simulink model "Step"  (R2018b)
settings: Solver=FixedStepDiscrete  StartTime=0.0  StopTime=10.0  RelTol=1e-3
libraries: simulink x5, vrlib x2
settings Model: Creator=taste  LastModifiedBy=taste
settings DataIOCC: SaveOutput=off  SignalLogging=off  SaveTime=off  ReturnWorkspaceOutputs=on
settings OptimizationCC: DefaultParameterBehavior=Inlined  EnhancedBackFolding=on  PassReuseOutputArgsAs=Individual arguments  ZeroExternalMemoryAtStartup=off  ZeroInternalMemoryAtStartup=off  OptimizeBlockOrder=speed  DifferentSizesBufferReuse=on  OptimizationCustomize=off
settings DebuggingCC: ParameterTunabilityLossMsg=error
settings SFSimCC: MATLABDynamicMemAlloc=off
settings RTWCC: SystemTargetFile=ert.tlc  TemplateMakefile=ert_default_tmf  PostCodeGenCommand=packNGo(buildInfo);
settings CodeAppCC: ForceParamTrailComments=on  IgnoreCustomStorageClasses=off  OperatorAnnotations=on  SimulinkDataObjDesc=on  SFDataObjDesc=on  InsertBlockDesc=on
settings ERTTargetCC: TargetLangStandard=C99 (ISO)  GenerateSampleERTMain=on  InlinedParameterPlacement=NonHierarchical  ERTCustomFileTemplate=example_file_process.tlc

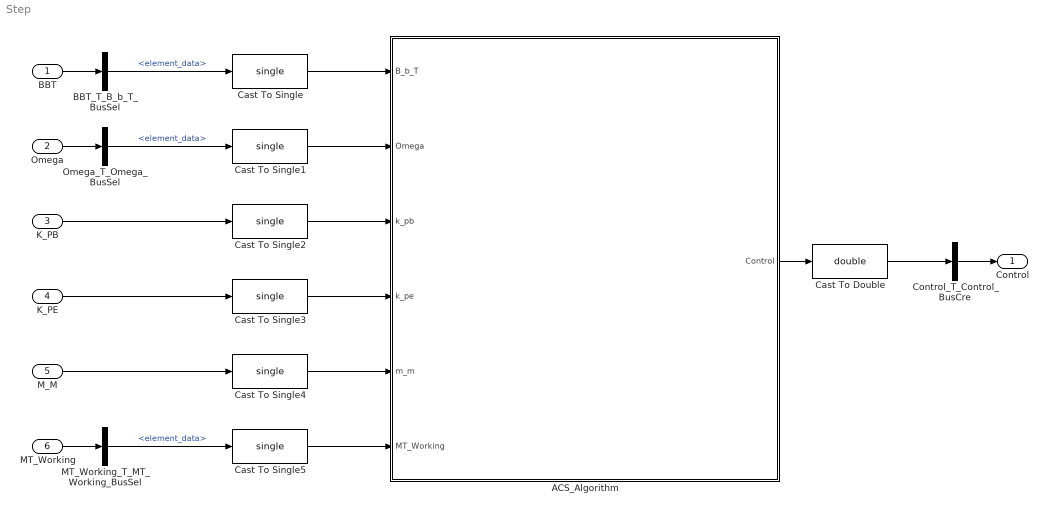
== system Step ==
  BBT : Inport  OutDataTypeStr=Bus: T_B_b_T  BusOutputAsStruct=on
  Omega : Inport  Port=2  OutDataTypeStr=Bus: T_Omega  BusOutputAsStruct=on
  K_PB : Inport  Port=3  OutDataTypeStr=T_Float  BusOutputAsStruct=on
  K_PE : Inport  Port=4  OutDataTypeStr=T_Float  BusOutputAsStruct=on
  M_M : Inport  Port=5  OutDataTypeStr=T_Float  BusOutputAsStruct=on
  MT_Working : Inport  Port=6  OutDataTypeStr=Bus: T_MT_Working  BusOutputAsStruct=on
  ACS_Algorithm : Subsystem
  BBT_T_B_b_T_BusSel : BusSelector  OutputSignals=element_data
  Cast To Double : DataTypeConversion  OutDataTypeStr=double
  Cast To Single{,1..5} (6 alike) : DataTypeConversion  OutDataTypeStr=single
  Control_T_Control_BusCre : BusCreator  Inputs=1  OutDataTypeStr=Bus: T_Control  NonVirtualBus=on
  MT_Working_T_MT_Working_BusSel : BusSelector  OutputSignals=element_data
  Omega_T_Omega_BusSel : BusSelector  OutputSignals=element_data
  Control : Outport  OutDataTypeStr=Bus: T_Control  BusOutputAsStruct=on
  wires:
  ACS_Algorithm/1(Control) -> Cast To Double/1
  Cast To Single/1 -> ACS_Algorithm/1(B_b_T)
  Cast To Single1/1 -> ACS_Algorithm/2(Omega)
  Cast To Single2/1 -> ACS_Algorithm/3(k_pb)
  Cast To Single3/1 -> ACS_Algorithm/4(k_pe)
  Cast To Single4/1 -> ACS_Algorithm/5(m_m)
  Cast To Single5/1 -> ACS_Algorithm/6(MT_Working)
  BBT/1 -> BBT_T_B_b_T_BusSel/1
  Omega/1 -> Omega_T_Omega_BusSel/1
  MT_Working/1 -> MT_Working_T_MT_Working_BusSel/1
  Control_T_Control_BusCre/1 -> Control/1
  BBT_T_B_b_T_BusSel/1 -> Cast To Single/1  "<element_data>"
  Omega_T_Omega_BusSel/1 -> Cast To Single1/1  "<element_data>"
  K_PB/1 -> Cast To Single2/1
  K_PE/1 -> Cast To Single3/1
  M_M/1 -> Cast To Single4/1
  MT_Working_T_MT_Working_BusSel/1 -> Cast To Single5/1  "<element_data>"
  Cast To Double/1 -> Control_T_Control_BusCre/1

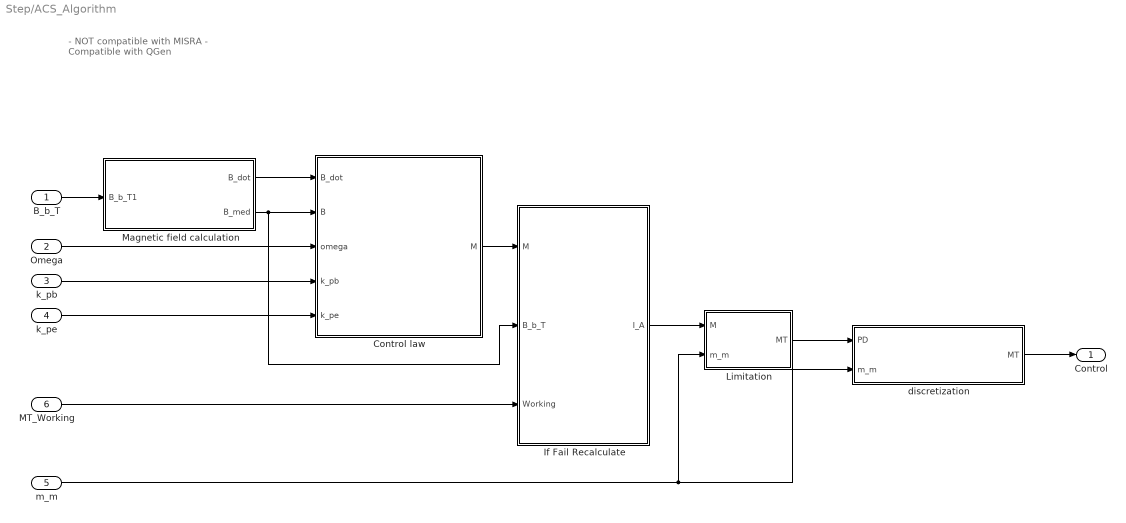
== system Step/ACS_Algorithm ==
  note: - NOT compatible with MISRA
      | - Compatible with QGen
  B_b_T : Inport  PortDimensions=15
  Omega : Inport  Port=2  PortDimensions=3
  k_pb : Inport  Port=3  PortDimensions=1
  k_pe : Inport  Port=4  PortDimensions=1
  m_m : Inport  Port=5  PortDimensions=1
  MT_Working : Inport  Port=6  PortDimensions=3
  Control law : Subsystem
  If Fail Recalculate : Subsystem
  Limitation : Subsystem
  Magnetic field calculation : Subsystem
  discretization : Subsystem
  Control : Outport  VectorParamsAs1DForOutWhenUnconnected=off
  wires:
  k_pb/1 -> Control law/4(k_pb)
  Magnetic field calculation/2(B_med) -> If Fail Recalculate/2(B_b_T), Control law/2(B)
  Omega/1 -> Control law/3(omega)
  Limitation/1(MT) -> discretization/1(PD)
  k_pe/1 -> Control law/5(k_pe)
  B_b_T/1 -> Magnetic field calculation/1(B_b_T1)
  If Fail Recalculate/1(I_A) -> Limitation/1(M)
  discretization/1(MT) -> Control/1
  Magnetic field calculation/1(B_dot) -> Control law/1(B_dot)
  m_m/1 -> Limitation/2(m_m), discretization/2(m_m)
  MT_Working/1 -> If Fail Recalculate/3(Working)
  Control law/1(M) -> If Fail Recalculate/1(M)

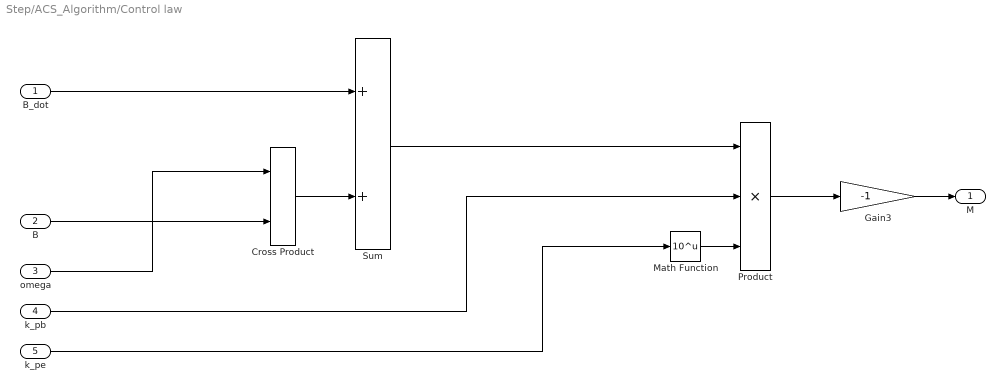
== system Step/ACS_Algorithm/Control law ==
  B_dot : Inport
  B : Inport  Port=2
  omega : Inport  Port=3
  k_pb : Inport  Port=4
  k_pe : Inport  Port=5
  Cross Product : vrlib/Utilities/Cross Product
  Gain3 : Gain  Gain=-1
  Math Function : Math  Operator=10^u  SaturateOnIntegerOverflow=on
  Product : Product  Inputs=3
  Sum : Sum  Inputs=2
  M : Outport  VectorParamsAs1DForOutWhenUnconnected=off
  wires:
  B/1 -> Cross Product/2
  Gain3/1 -> M/1
  Sum/1 -> Product/1
  B_dot/1 -> Sum/1
  Cross Product/1 -> Sum/2
  Product/1 -> Gain3/1
  Math Function/1 -> Product/3
  k_pb/1 -> Product/2
  k_pe/1 -> Math Function/1
  omega/1 -> Cross Product/1

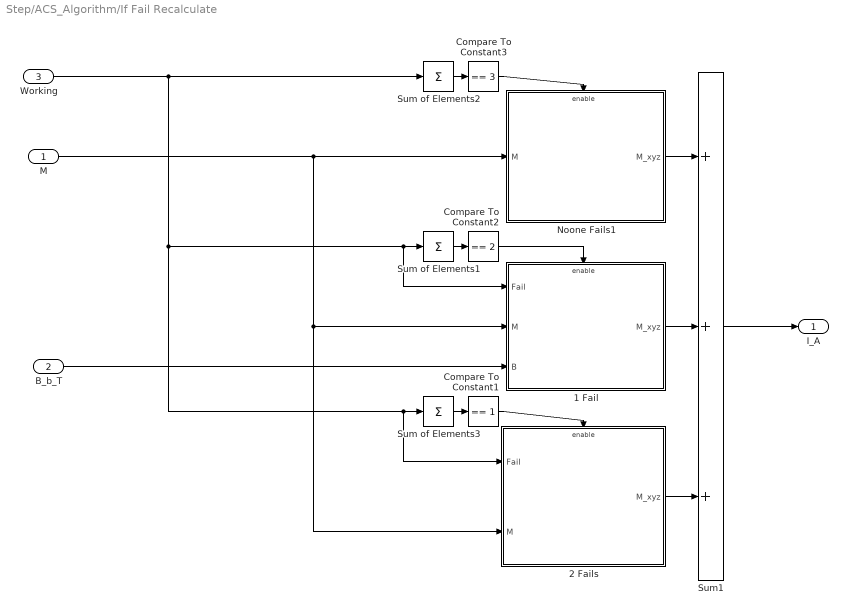
== system Step/ACS_Algorithm/If Fail Recalculate ==
  M : Inport
  B_b_T : Inport  Port=2
  Working : Inport  Port=3
  1 Fail : Subsystem
  2 Fails : Subsystem
  Compare To Constant1 : simulink/Logic and Bit Operations/Compare To Constant  relop===  const=1  OutDataTypeStr=uint8  ZeroCross=off
  Compare To Constant2 : simulink/Logic and Bit Operations/Compare To Constant  relop===  const=2  OutDataTypeStr=uint8  ZeroCross=off
  Compare To Constant3 : simulink/Logic and Bit Operations/Compare To Constant  relop===  const=3  OutDataTypeStr=uint8  ZeroCross=off
  Noone Fails1 : Subsystem
  Sum of Elements1 : Sum  Inputs=+
  Sum of Elements2 : Sum  Inputs=+
  Sum of Elements3 : Sum  Inputs=+
  Sum1 : Sum  Inputs=3
  I_A : Outport  VectorParamsAs1DForOutWhenUnconnected=off
  wires:
  Compare To Constant1/1 -> 2 Fails/Enable
  2 Fails/1(M_xyz) -> Sum1/3
  Sum of Elements3/1 -> Compare To Constant1/1
  Sum of Elements2/1 -> Compare To Constant3/1
  Sum of Elements1/1 -> Compare To Constant2/1
  M/1 -> 2 Fails/2(M), 1 Fail/2(M), Noone Fails1/1(M)
  Compare To Constant2/1 -> 1 Fail/Enable
  Compare To Constant3/1 -> Noone Fails1/Enable
  1 Fail/1(M_xyz) -> Sum1/2
  Noone Fails1/1(M_xyz) -> Sum1/1
  B_b_T/1 -> 1 Fail/3(B)
  Working/1 -> Sum of Elements2/1, 2 Fails/1(Fail), Sum of Elements3/1, 1 Fail/1(Fail), Sum of Elements1/1
  Sum1/1 -> I_A/1

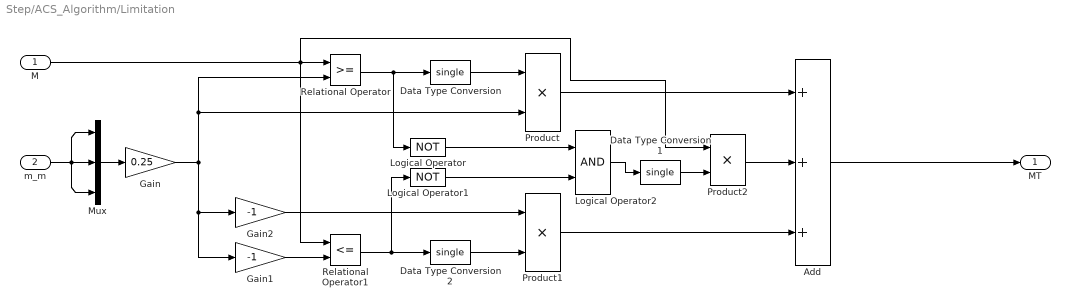
== system Step/ACS_Algorithm/Limitation ==
  M : Inport
  m_m : Inport  Port=2
  Add : Sum  Inputs=3
  Data Type Conversion : DataTypeConversion  OutDataTypeStr=single
  Data Type Conversion1 : DataTypeConversion  OutDataTypeStr=single
  Data Type Conversion2 : DataTypeConversion  OutDataTypeStr=single
  Gain : Gain  Gain=0.25
  Gain1 : Gain  Gain=-1
  Gain2 : Gain  Gain=-1
  Logical Operator : Logic  Operator=NOT  AllPortsSameDT=off  OutDataTypeStr=boolean
  Logical Operator1 : Logic  Operator=NOT  AllPortsSameDT=off  OutDataTypeStr=boolean
  Logical Operator2 : Logic  AllPortsSameDT=off  OutDataTypeStr=boolean
  Mux : Mux  Inputs=3
  Product : Product
  Product1 : Product
  Product2 : Product
  Relational Operator : RelationalOperator  OutDataTypeStr=boolean  RndMeth=Nearest
  Relational Operator1 : RelationalOperator  Operator=<=  OutDataTypeStr=boolean  RndMeth=Nearest
  MT : Outport  VectorParamsAs1DForOutWhenUnconnected=off
  wires:
  M/1 -> Product2/1, Relational Operator1/1, Relational Operator/1
  m_m/1 -> Mux/3, Mux/1, Mux/2
  Gain/1 -> Relational Operator/2, Product/2, Gain2/1, Gain1/1
  Gain1/1 -> Relational Operator1/2
  Relational Operator/1 -> Logical Operator/1, Data Type Conversion/1
  Relational Operator1/1 -> Logical Operator1/1, Data Type Conversion2/1
  Logical Operator/1 -> Logical Operator2/1
  Logical Operator1/1 -> Logical Operator2/2
  Logical Operator2/1 -> Data Type Conversion1/1
  Product/1 -> Add/1
  Product2/1 -> Add/2
  Product1/1 -> Add/3
  Gain2/1 -> Product1/1
  Mux/1 -> Gain/1
  Add/1 -> MT/1
  Data Type Conversion/1 -> Product/1
  Data Type Conversion1/1 -> Product2/2
  Data Type Conversion2/1 -> Product1/2

== system Step/ACS_Algorithm/Magnetic field calculation ==
  B_b_T1 : Inport
  Derivative : Subsystem
  Media : Subsystem
  B_dot : Outport  VectorParamsAs1DForOutWhenUnconnected=off
  B_med : Outport  Port=2  VectorParamsAs1DForOutWhenUnconnected=off
  wires:
  B_b_T1/1 -> Derivative/1(In1), Media/1(B_b_T_1s)
  Media/1(B_b_T_1s_m) -> B_med/1
  Derivative/1(B_dot) -> B_dot/1

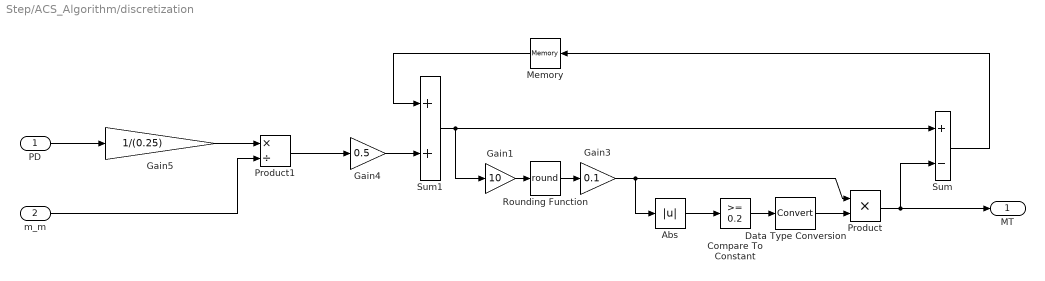
== system Step/ACS_Algorithm/discretization ==
  PD : Inport
  m_m : Inport  Port=2
  Abs : Abs
  Compare To Constant : simulink/Logic and Bit Operations/Compare To Constant  relop=>=  const=0.2  OutDataTypeStr=uint8  ZeroCross=off
  Data Type Conversion : DataTypeConversion
  Gain1 : Gain  Gain=10
  Gain3 : Gain  Gain=0.1
  Gain4 : Gain  Gain=0.5
  Gain5 : Gain  Gain=1/(0.25)
  Memory : Memory  InheritSampleTime=on
  Product : Product  RndMeth=Zero
  Product1 : Product  Inputs=*/  RndMeth=Zero
  Rounding Function : Rounding  Operator=round
  Sum : Sum  Inputs=+-
  Sum1 : Sum  Inputs=2
  MT : Outport  VectorParamsAs1DForOutWhenUnconnected=off
  wires:
  Rounding Function/1 -> Gain3/1
  Gain1/1 -> Rounding Function/1
  Sum/1 -> Memory/1
  Sum1/1 -> Gain1/1, Sum/1
  Gain3/1 -> Abs/1, Product/1
  Compare To Constant/1 -> Data Type Conversion/1
  Data Type Conversion/1 -> Product/2
  Abs/1 -> Compare To Constant/1
  PD/1 -> Gain5/1
  Product/1 -> MT/1, Sum/2
  Memory/1 -> Sum1/1
  Gain4/1 -> Sum1/2
  Gain5/1 -> Product1/1
  Product1/1 -> Gain4/1
  m_m/1 -> Product1/2

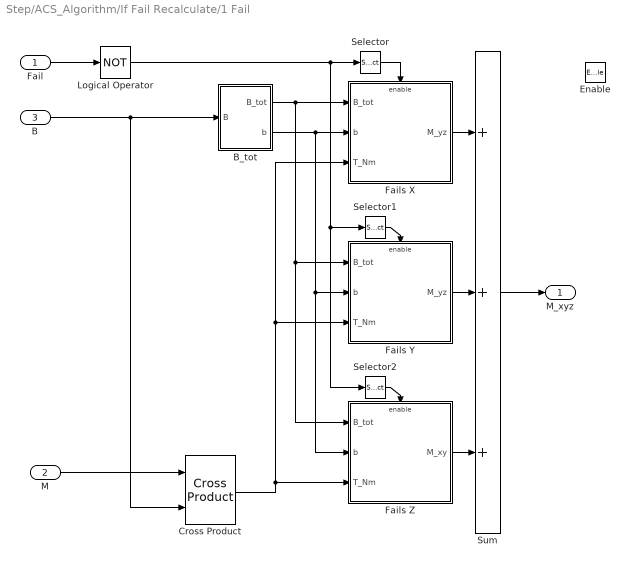
== system Step/ACS_Algorithm/If Fail Recalculate/1 Fail ==
  Fail : Inport
  M : Inport  Port=2
  B : Inport  Port=3
  Enable : EnablePort
  B_tot : Subsystem
  Cross Product : vrlib/Utilities/Cross Product
  Fails X : Subsystem
  Fails Y : Subsystem
  Fails Z : Subsystem
  Logical Operator : Logic  Operator=NOT  AllPortsSameDT=off  OutDataTypeStr=boolean
  Selector : Selector  InputPortWidth=3  IndexOptions=Index vector (dialog)  Indices=[1]  OutputSizes=1
  Selector1 : Selector  InputPortWidth=3  IndexOptions=Index vector (dialog)  Indices=[2]  OutputSizes=1
  Selector2 : Selector  InputPortWidth=3  IndexOptions=Index vector (dialog)  Indices=[3]  OutputSizes=1
  Sum : Sum  Inputs=3
  M_xyz : Outport  VectorParamsAs1DForOutWhenUnconnected=off
  wires:
  Sum/1 -> M_xyz/1
  M/1 -> Cross Product/1
  B/1 -> Cross Product/2, B_tot/1(B)
  B_tot/1(B_tot) -> Fails X/1(B_tot), Fails Y/1(B_tot), Fails Z/1(B_tot)
  B_tot/2(b) -> Fails Y/2(b), Fails Z/2(b), Fails X/2(b)
  Cross Product/1 -> Fails X/3(T_Nm), Fails Y/3(T_Nm), Fails Z/3(T_Nm)
  Fails X/1(M_yz) -> Sum/1
  Fails Y/1(M_yz) -> Sum/2
  Fails Z/1(M_xy) -> Sum/3
  Selector/1 -> Fails X/Enable
  Selector1/1 -> Fails Y/Enable
  Selector2/1 -> Fails Z/Enable
  Fail/1 -> Logical Operator/1
  Logical Operator/1 -> Selector/1, Selector1/1, Selector2/1

== system Step/ACS_Algorithm/If Fail Recalculate/2 Fails ==
  Fail : Inport
  M : Inport  Port=2
  Enable : EnablePort
  Demux1 : Demux  Outputs=3
  Demux3 : Demux  Outputs=3
  Mux : Mux  Inputs=3
  Product : Product  RndMeth=Zero
  Product1 : Product  RndMeth=Zero
  Product2 : Product  RndMeth=Zero
  M_xyz : Outport  VectorParamsAs1DForOutWhenUnconnected=off
  wires:
  Mux/1 -> M_xyz/1
  M/1 -> Demux3/1
  Product2/1 -> Mux/3
  Product1/1 -> Mux/2
  Product/1 -> Mux/1
  Demux3/1 -> Product/1
  Demux3/2 -> Product1/1
  Demux3/3 -> Product2/1
  Demux1/3 -> Product2/2
  Demux1/2 -> Product1/2
  Fail/1 -> Demux1/1
  Demux1/1 -> Product/2

== system Step/ACS_Algorithm/If Fail Recalculate/Noone Fails1 ==
  M : Inport
  Enable : EnablePort
  M_xyz : Outport  VectorParamsAs1DForOutWhenUnconnected=off
  wires:
  M/1 -> M_xyz/1

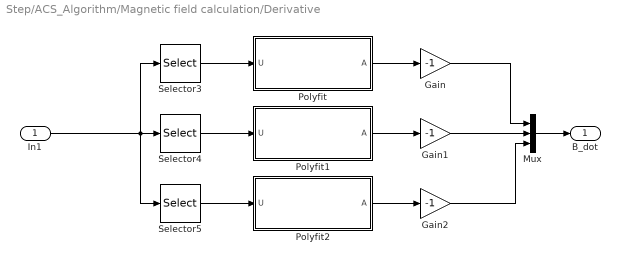
== system Step/ACS_Algorithm/Magnetic field calculation/Derivative ==
  In1 : Inport
  Gain : Gain  Gain=-1
  Gain1 : Gain  Gain=-1
  Gain2 : Gain  Gain=-1
  Mux : Mux  Inputs=3
  Polyfit : Subsystem
  Polyfit1 : Subsystem
  Polyfit2 : Subsystem
  Selector3 : Selector  InputPortWidth=15  IndexOptions=Index vector (dialog)  Indices=[1 4 7 10 13]  OutputSizes=1
  Selector4 : Selector  InputPortWidth=15  IndexOptions=Index vector (dialog)  Indices=[2 5 8 11 14]  OutputSizes=1
  Selector5 : Selector  InputPortWidth=15  IndexOptions=Index vector (dialog)  Indices=[3 6 9 12 15]  OutputSizes=1
  B_dot : Outport  VectorParamsAs1DForOutWhenUnconnected=off
  wires:
  In1/1 -> Selector3/1, Selector4/1, Selector5/1
  Mux/1 -> B_dot/1
  Gain/1 -> Mux/1
  Gain1/1 -> Mux/2
  Gain2/1 -> Mux/3
  Selector3/1 -> Polyfit/1(U)
  Selector4/1 -> Polyfit1/1(U)
  Selector5/1 -> Polyfit2/1(U)
  Polyfit/1(A) -> Gain/1
  Polyfit1/1(A) -> Gain1/1
  Polyfit2/1(A) -> Gain2/1

== system Step/ACS_Algorithm/Magnetic field calculation/Media ==
  B_b_T_1s : Inport
  Demux : Demux  Outputs=5
  Gain : Gain  Gain=1/5
  Sum1 : Sum  Inputs=5
  B_b_T_1s_m : Outport  VectorParamsAs1DForOutWhenUnconnected=off
  wires:
  Sum1/1 -> Gain/1
  Gain/1 -> B_b_T_1s_m/1
  B_b_T_1s/1 -> Demux/1
  Demux/1 -> Sum1/1
  Demux/2 -> Sum1/2
  Demux/3 -> Sum1/3
  Demux/4 -> Sum1/4
  Demux/5 -> Sum1/5

== system Step/ACS_Algorithm/If Fail Recalculate/1 Fail/B_tot ==
  B : Inport
  Subsystem : Subsystem
  B_tot : Outport  VectorParamsAs1DForOutWhenUnconnected=off
  b : Outport  Port=2  VectorParamsAs1DForOutWhenUnconnected=off
  wires:
  B/1 -> Subsystem/1(B)
  Subsystem/1(B_tot) -> B_tot/1
  Subsystem/2(b) -> b/1

== system Step/ACS_Algorithm/If Fail Recalculate/1 Fail/Fails X ==
  B_tot : Inport
  b : Inport  Port=2
  T_Nm : Inport  Port=3
  Enable : EnablePort
  Constant : Constant  Value=0  OutDataTypeStr=single
  Matrix x-fails : Subsystem
  Mux : Mux  Inputs=2
  Product1 : Product  Multiplication=Matrix(*)  RndMeth=Zero
  Product3 : Product  Inputs=/*  RndMeth=Zero
  M_yz : Outport  VectorParamsAs1DForOutWhenUnconnected=off
  wires:
  Matrix x-fails/1(M2) -> Product1/1
  T_Nm/1 -> Product1/2
  Product1/1 -> Product3/2
  Product3/1 -> Mux/2
  Mux/1 -> M_yz/1
  B_tot/1 -> Product3/1
  b/1 -> Matrix x-fails/1(b)
  Constant/1 -> Mux/1

== system Step/ACS_Algorithm/If Fail Recalculate/1 Fail/Fails Y ==
  B_tot : Inport
  b : Inport  Port=2
  T_Nm : Inport  Port=3
  Enable : EnablePort
  Constant : Constant  Value=0  OutDataTypeStr=single
  Demux : Demux  Outputs=2
  Matrix y-fails : Subsystem
  Mux : Mux  Inputs=3
  Product1 : Product  Multiplication=Matrix(*)  RndMeth=Zero
  Product3 : Product  Inputs=/*  RndMeth=Zero
  M_yz : Outport  VectorParamsAs1DForOutWhenUnconnected=off
  wires:
  b/1 -> Matrix y-fails/1(b)
  B_tot/1 -> Product3/1
  Mux/1 -> M_yz/1
  Product1/1 -> Product3/2
  T_Nm/1 -> Product1/2
  Matrix y-fails/1(M2) -> Product1/1
  Product3/1 -> Demux/1
  Demux/1 -> Mux/1
  Demux/2 -> Mux/3
  Constant/1 -> Mux/2

== system Step/ACS_Algorithm/If Fail Recalculate/1 Fail/Fails Z ==
  B_tot : Inport
  b : Inport  Port=2
  T_Nm : Inport  Port=3
  Enable : EnablePort
  Constant : Constant  Value=0  OutDataTypeStr=single
  Matrix z-fails : Subsystem
  Mux : Mux  Inputs=2
  Product1 : Product  Multiplication=Matrix(*)  RndMeth=Zero
  Product3 : Product  Inputs=/*  RndMeth=Zero
  M_xy : Outport  VectorParamsAs1DForOutWhenUnconnected=off
  wires:
  Matrix z-fails/1(M2) -> Product1/1
  T_Nm/1 -> Product1/2
  Product1/1 -> Product3/2
  Mux/1 -> M_xy/1
  B_tot/1 -> Product3/1
  b/1 -> Matrix z-fails/1(b)
  Product3/1 -> Mux/1
  Constant/1 -> Mux/2

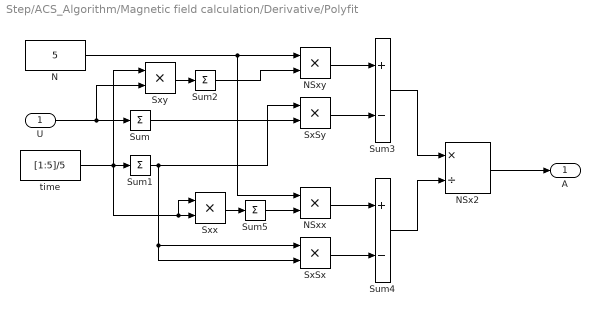
== system Step/ACS_Algorithm/Magnetic field calculation/Derivative/Polyfit ==
  U : Inport
  N : Constant  Value=5  OutDataTypeStr=single
  NSx2 : Product  Inputs=*/
  NSxx : Product
  NSxy : Product
  Sum{,1..2,5} (4 alike) : Sum  Inputs=+
  Sum3 : Sum  Inputs=+-
  Sum4 : Sum  Inputs=+-
  SxSx : Product
  "SxSy " : Product
  Sxx : Product
  Sxy : Product
  time : Constant  Value=[1:5]/5  OutDataTypeStr=single
  A : Outport  VectorParamsAs1DForOutWhenUnconnected=off
  wires:
  U/1 -> Sxy/2, Sum/1
  time/1 -> Sxx/2, Sxx/1, Sxy/1, Sum1/1
  N/1 -> NSxx/1, NSxy/1
  Sxy/1 -> Sum2/1
  NSxy/1 -> Sum3/1
  Sum1/1 -> SxSx/2, SxSx/1, "SxSy "/1
  Sum/1 -> "SxSy "/2
  "SxSy "/1 -> Sum3/2
  NSx2/1 -> A/1
  Sxx/1 -> Sum5/1
  NSxx/1 -> Sum4/1
  SxSx/1 -> Sum4/2
  Sum3/1 -> NSx2/1
  Sum4/1 -> NSx2/2
  Sum2/1 -> NSxy/2
  Sum5/1 -> NSxx/2

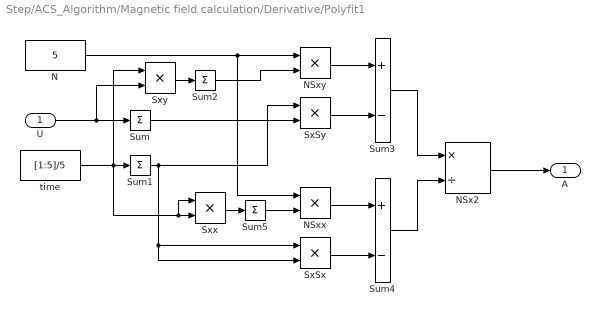
== system Step/ACS_Algorithm/Magnetic field calculation/Derivative/Polyfit1 ==
  U : Inport
  N : Constant  Value=5  OutDataTypeStr=single
  NSx2 : Product  Inputs=*/
  NSxx : Product
  NSxy : Product
  Sum{,1..2,5} (4 alike) : Sum  Inputs=+
  Sum3 : Sum  Inputs=+-
  Sum4 : Sum  Inputs=+-
  SxSx : Product
  "SxSy " : Product
  Sxx : Product
  Sxy : Product
  time : Constant  Value=[1:5]/5  OutDataTypeStr=single
  A : Outport  VectorParamsAs1DForOutWhenUnconnected=off
  wires:
  Sum5/1 -> NSxx/2
  Sum2/1 -> NSxy/2
  Sum4/1 -> NSx2/2
  Sum3/1 -> NSx2/1
  SxSx/1 -> Sum4/2
  NSxx/1 -> Sum4/1
  Sxx/1 -> Sum5/1
  NSx2/1 -> A/1
  "SxSy "/1 -> Sum3/2
  Sum/1 -> "SxSy "/2
  Sum1/1 -> "SxSy "/1, SxSx/1, SxSx/2
  NSxy/1 -> Sum3/1
  Sxy/1 -> Sum2/1
  N/1 -> NSxy/1, NSxx/1
  time/1 -> Sum1/1, Sxy/1, Sxx/1, Sxx/2
  U/1 -> Sum/1, Sxy/2

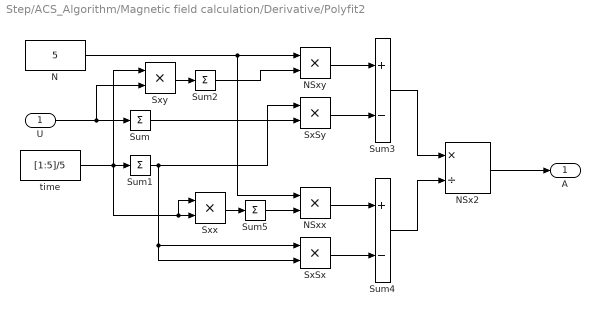
== system Step/ACS_Algorithm/Magnetic field calculation/Derivative/Polyfit2 ==
  U : Inport
  N : Constant  Value=5  OutDataTypeStr=single
  NSx2 : Product  Inputs=*/
  NSxx : Product
  NSxy : Product
  Sum{,1..2,5} (4 alike) : Sum  Inputs=+
  Sum3 : Sum  Inputs=+-
  Sum4 : Sum  Inputs=+-
  SxSx : Product
  "SxSy " : Product
  Sxx : Product
  Sxy : Product
  time : Constant  Value=[1:5]/5  OutDataTypeStr=single
  A : Outport  VectorParamsAs1DForOutWhenUnconnected=off
  wires:
  U/1 -> Sxy/2, Sum/1
  time/1 -> Sxx/2, Sxx/1, Sxy/1, Sum1/1
  N/1 -> NSxx/1, NSxy/1
  Sxy/1 -> Sum2/1
  NSxy/1 -> Sum3/1
  Sum1/1 -> SxSx/2, SxSx/1, "SxSy "/1
  Sum/1 -> "SxSy "/2
  "SxSy "/1 -> Sum3/2
  NSx2/1 -> A/1
  Sxx/1 -> Sum5/1
  NSxx/1 -> Sum4/1
  SxSx/1 -> Sum4/2
  Sum3/1 -> NSx2/1
  Sum4/1 -> NSx2/2
  Sum2/1 -> NSxy/2
  Sum5/1 -> NSxx/2

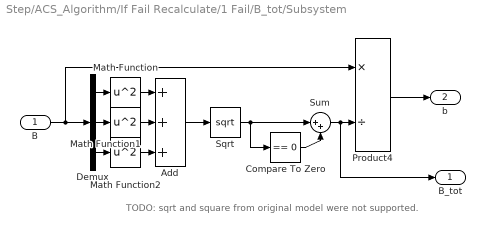
== system Step/ACS_Algorithm/If Fail Recalculate/1 Fail/B_tot/Subsystem ==
  note: TODO: sqrt and square from original model were not supported.
  B : Inport
  Add : Sum  Inputs=+++
  Compare To Zero : simulink/Logic and Bit Operations/Compare To Zero  relop===  OutDataTypeStr=uint8  ZeroCross=off
  Demux : Demux  Outputs=3
  Math Function : Math  Operator=square  SaturateOnIntegerOverflow=on
  Math Function1 : Math  Operator=square  SaturateOnIntegerOverflow=on
  Math Function2 : Math  Operator=square  SaturateOnIntegerOverflow=on
  Product4 : Product  Inputs=*/  RndMeth=Zero
  Sqrt : Sqrt  IntermediateResultsDataTypeStr=double  SaturateOnIntegerOverflow=on
  Sum : Sum  Inputs=|++
  B_tot : Outport  VectorParamsAs1DForOutWhenUnconnected=off
  b : Outport  Port=2  VectorParamsAs1DForOutWhenUnconnected=off
  wires:
  Demux/2 -> Math Function1/1
  Demux/1 -> Math Function/1
  B/1 -> Demux/1, Product4/1
  Demux/3 -> Math Function2/1
  Sqrt/1 -> Compare To Zero/1, Sum/1
  Math Function/1 -> Add/1
  Product4/1 -> b/1
  Math Function1/1 -> Add/2
  Add/1 -> Sqrt/1
  Compare To Zero/1 -> Sum/2
  Math Function2/1 -> Add/3
  Sum/1 -> B_tot/1, Product4/2

== system Step/ACS_Algorithm/If Fail Recalculate/1 Fail/Fails X/Matrix x-fails ==
  b : Inport
  Fcn10 : Fcn  Expr=(1-u(2)^2)/(u(1)+1e-10*(u(1)==0))
  Fcn5 : Fcn  Expr=(u(3))
  Fcn6 : Fcn  Expr=-(u(2))
  Fcn7 : Fcn  Expr=(u(2)*u(3))/(u(1)+1e-10*(u(1)==0))
  Fcn8 : Fcn  Expr=-(u(2)*u(3))/(u(1)+1e-10*(u(1)==0))
  Fcn9 : Fcn  Expr=-(1-u(3)^2)/(u(1)+1e-10*(u(1)==0))
  Mux : Mux  Inputs=6
  Reshape : Reshape  OutputDimensionality=Customize  OutputDimensions=[2,3]
  M2 : Outport  VectorParamsAs1DForOutWhenUnconnected=off
  wires:
  Fcn5/1 -> Mux/1
  b/1 -> Fcn5/1, Fcn6/1, Fcn10/1, Fcn9/1, Fcn8/1, Fcn7/1
  Reshape/1 -> M2/1
  Mux/1 -> Reshape/1
  Fcn6/1 -> Mux/2
  Fcn7/1 -> Mux/3
  Fcn8/1 -> Mux/6
  Fcn10/1 -> Mux/4
  Fcn9/1 -> Mux/5

== system Step/ACS_Algorithm/If Fail Recalculate/1 Fail/Fails Y/Matrix y-fails ==
  b : Inport
  Fcn1 : Fcn  Expr=(u(1)*u(3))/(u(2)+1e-10*(u(2)==0))
  Fcn2 : Fcn  Expr=(1-u(3)^2)/(u(2)+1e-10*(u(2)==0))
  Fcn3 : Fcn  Expr=(u(1))
  Fcn5 : Fcn  Expr=-(u(3))
  Fcn8 : Fcn  Expr=-(u(1)*u(3))/(u(2)+1e-10*(u(2)==0))
  Fcn9 : Fcn  Expr=-(1-u(1)^2)/(u(2)+1e-10*(u(2)==0))
  Mux : Mux  Inputs=6
  Reshape : Reshape  OutputDimensionality=Customize  OutputDimensions=[2,3]
  M2 : Outport  VectorParamsAs1DForOutWhenUnconnected=off
  wires:
  Fcn2/1 -> Mux/5
  Fcn3/1 -> Mux/4
  Fcn1/1 -> Mux/6
  Fcn5/1 -> Mux/3
  Mux/1 -> Reshape/1
  Reshape/1 -> M2/1
  b/1 -> Fcn1/1, Fcn2/1, Fcn3/1, Fcn5/1, Fcn8/1, Fcn9/1
  Fcn9/1 -> Mux/2
  Fcn8/1 -> Mux/1

== system Step/ACS_Algorithm/If Fail Recalculate/1 Fail/Fails Z/Matrix z-fails ==
  b : Inport
  Fcn1 : Fcn  Expr=-(u(2)*u(1))/(u(3)+1e-10*(u(3)==0))
  Fcn10 : Fcn  Expr=(1-u(1)^2)/(u(3)+1e-10*(u(3)==0))
  Fcn2 : Fcn  Expr=-(u(1))
  Fcn3 : Fcn  Expr=-(1-u(2)^2)/(u(3)+1e-10*(u(3)==0))
  Fcn6 : Fcn  Expr=(u(2))
  Fcn7 : Fcn  Expr=(u(2)*u(1))/(u(3)+1e-10*(u(3)==0))
  Mux : Mux  Inputs=6
  Reshape : Reshape  OutputDimensionality=Customize  OutputDimensions=[2,3]
  M2 : Outport  VectorParamsAs1DForOutWhenUnconnected=off
  wires:
  b/1 -> Fcn7/1, Fcn10/1, Fcn6/1, Fcn2/1, Fcn1/1, Fcn3/1
  Reshape/1 -> M2/1
  Mux/1 -> Reshape/1
  Fcn3/1 -> Mux/3
  Fcn2/1 -> Mux/6
  Fcn1/1 -> Mux/4
  Fcn6/1 -> Mux/5
  Fcn7/1 -> Mux/1
  Fcn10/1 -> Mux/2
